simulink model "nmreflex_step"  (R2014a)
settings: Solver=ode3  SolverMode=SingleTasking  StartTime=0.0  StopTime=100  FixedStep=0.001  MaxStep=0.001  RelTol=1e-3  AbsTol=1e-3
values from neighbouring files (symbols this model uses):
  B = 1    [nmr_var.m]    (also in questao3.m = 2; questao5b.m = 2)
  beta = 50    [nmr_var.m]    (also in questao3.m = 100; questao5b.m = iBeta)
  eta = 5    [nmr_var.m]    (also in questao3.m; questao5b.m)
  J = 0.1    [nmr_var.m]    (also in questao3.m; questao5b.m)
  k = 50    [nmr_var.m]    (also in nyqlog.m = 1; questao3.m; questao5b.m)
  tau = 1/300    (= 0.00333333333333)    [nmr_var.m]    (also in questao3.m; questao5b.m)
  Td = 0.02    [nmr_var.m]    (also in questao3.m = 0; questao5b.m = dValues(iD))
settings Model: Creator=Administrator  LastModifiedBy=Andre
settings DataIOCC: LimitDataPoints=off  SaveOutput=off  SaveTime=off  SignalLoggingName=sigsOut
settings OptimizationCC: BooleanDataType=off  ExpressionDepthLimit=2147483647  InitFltsAndDblsToZero=on
settings DebuggingCC: SaveWithParameterizedLinksMsg=none  UnderspecifiedInitializationDetection=Classic  SignalResolutionControl=TryResolveAllWithWarning  SolverPrmCheckMsg=none  MultiTaskDSMMsg=warning  MultiTaskCondExecSysMsg=none  StateNameClashWarn=warning
settings HardwareCC: TargetUnknown=on
settings RTWCC: TemplateMakefile=grt_vc.tmf  IncludeERTFirstTime=on
settings GRTTargetCC: TargetFcnLib=ansi_tfl_tmw.mat  CombineOutputUpdateFcns=off  GRTInterface=on

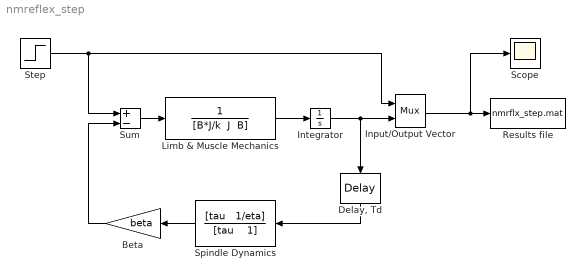
== system nmreflex_step ==
  Beta : Gain  Gain=beta  SaturateOnIntegerOverflow=on  OutDataTypeStr=Inherit: Same as input  ParamDataTypeStr=Inherit: Same as input
  "Delay, Td " : TransportDelay  DelayTime=Td
  Input/Output Vector : Mux  Inputs=2
  Integrator : Integrator
  Limb & Muscle Mechanics : TransferFcn  Denominator="[B*J/k  J  B]"
  Results file : ToFile  Filename=nmrflx_step.mat  MatrixName=result
  Scope : Scope
      settings: TickLabels=on  TimeRange=6  YMin=-1  YMax=1  MaxDataPoints=200000
  Spindle Dynamics : TransferFcn  Numerator="[tau   1/eta]"  Denominator="[tau    1]"
  Step : Step  SampleTime=0
  Sum : Sum  Inputs=+-  SaturateOnIntegerOverflow=on  InputSameDT=on  OutDataTypeStr=Inherit: Same as first input
  wires:
  Limb & Muscle Mechanics/1 -> Integrator/1
  Spindle Dynamics/1 -> Beta/1
  Sum/1 -> Limb & Muscle Mechanics/1
  "Delay, Td "/1 -> Spindle Dynamics/1
  Integrator/1 -> Input/Output Vector/2, "Delay, Td "/1
  Beta/1 -> Sum/2
  Step/1 -> Sum/1, Input/Output Vector/1
  Input/Output Vector/1 -> Scope/1, Results file/1
